simulink model "AutopilotLinear"  (R2021a)
settings: Solver=VariableStepAuto  StartTime=0.0  StopTime=2500  RelTol=1e-3
values from neighbouring files (symbols this model uses):
  A_final = [A1_long,zeros(5);zeros(5),A1_latr]    [runMeFirst.m]
  B_final = [B1_long,zeros(5,2);zeros(5,2),B1_latr]    [runMeFirst.m]
  C_final = [C1_long,zeros(5);zeros(5),C1_latr]    [runMeFirst.m]
  D_final = zeros(10,4)    [runMeFirst.m]
  Initial_h = 1000    [runMeFirst.m]
  K_deltas = [K_deltas_long,zeros(2);zeros(2),K_deltas_latr]    [runMeFirst.m]
  K_eps = [K_eps_long,zeros(2,2);zeros(2,2),K_eps_latr]    [runMeFirst.m]
  K_lqr = [K_lqr_long,zeros(2,5);zeros(2,5),K_lqr_latr]    [runMeFirst.m]
  Second_h = 2000    [runMeFirst.m]
  Start_time = 500    [runMeFirst.m]
  Start_turn = 1500    [runMeFirst.m]
  Step_timeh = 1000    [runMeFirst.m]
  T_a = 0.0495    [Auto_latr2.mat]
  T_e = 0.1    [Auto_long2.mat]
  T_p = 3.5    [Auto_long2.mat]
  T_r = 0.0495    [Auto_latr2.mat]
  Ue = 67    [runMeFirst.m]
undefined symbols (not defined in the file or in its folder): Des_rate, Des_roll
libraries: aerolibconvert2 x5, simulink x2
settings Model: Creator=panch  LastModifiedBy=panch

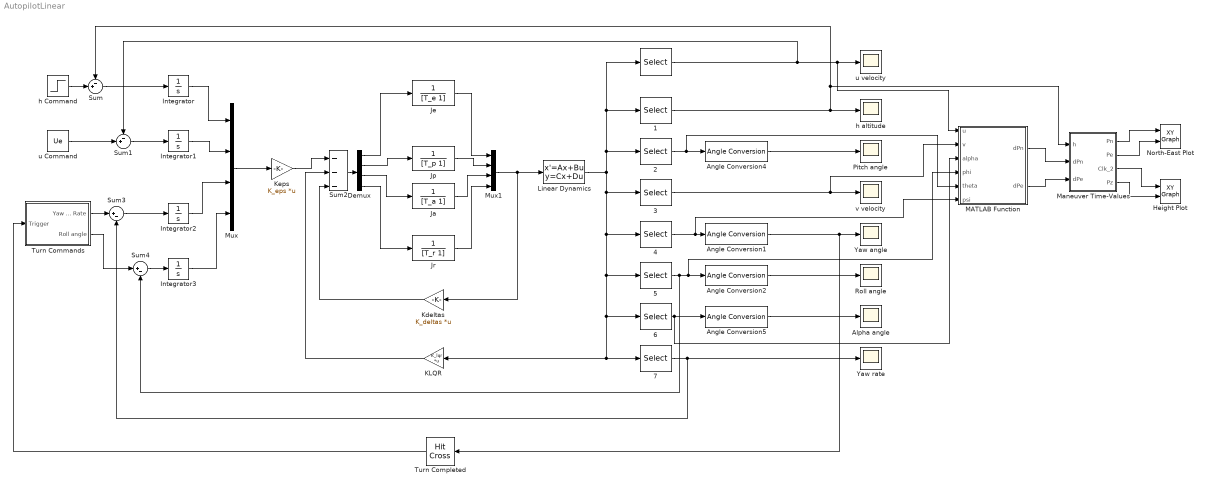
== system AutopilotLinear ==
  " " : Selector  InputPortWidth=10  IndexOptions=Index vector (dialog)  Indices=1  OutputSizes=1
  " 1" : Selector  InputPortWidth=10  IndexOptions=Index vector (dialog)  Indices=5  OutputSizes=1
  " 2" : Selector  InputPortWidth=10  IndexOptions=Index vector (dialog)  Indices=4  OutputSizes=1
  " 3" : Selector  InputPortWidth=10  IndexOptions=Index vector (dialog)  Indices=6  OutputSizes=1
  " 4" : Selector  InputPortWidth=10  IndexOptions=Index vector (dialog)  Indices=10  OutputSizes=1
  " 5" : Selector  InputPortWidth=10  IndexOptions=Index vector (dialog)  Indices=9  OutputSizes=1
  " 6" : Selector  InputPortWidth=10  IndexOptions=Index vector (dialog)  Indices=2  OutputSizes=1
  " 7" : Selector  InputPortWidth=10  IndexOptions=Index vector (dialog)  Indices=8  OutputSizes=1
  Alpha angle : Scope
  Angle Conversion{1..2,4..5} (4 alike) : aerolibconvert2/Angle Conversion  IU=rad  OU=deg
  Demux : Demux
  Height Plot : simulink/Sinks/XY Graph  xmin=0  xmax=2000  ymin=0  ymax=2500  st=-1
  Integrator{,1..3} (4 alike) : Integrator
  Ja : TransferFcn  Denominator=[T_a 1]
  Je : TransferFcn  Denominator=[T_e 1]
  Jp : TransferFcn  Denominator=[T_p 1]
  Jr : TransferFcn  Denominator=[T_r 1]
  KLQR : Gain  Gain=K_lqr  Multiplication=Matrix(K*u)
  Kdeltas : Gain  Gain=K_deltas  Multiplication=Matrix(K*u)
  Keps : Gain  Gain=K_eps  Multiplication=Matrix(K*u)
  Linear Dynamics : StateSpace  A=A_final  B=B_final  C=C_final  D=D_final  InitialCondition=0
  MATLAB Function : MATLAB Function  TreatAsAtomicUnit=on
  Maneuver Time-Values : Subsystem
  Mux : Mux
  Mux1 : Mux
  North-East Plot : simulink/Sinks/XY Graph  xmin=0  xmax=0.7e5  ymin=-100  ymax=4500  st=-1
  Pitch angle : Scope
  Roll angle : Scope
  Sum : Sum  Inputs=-+|
  Sum1 : Sum  Inputs=-+|
  Sum2 : Sum  Inputs=|---
  Sum3 : Sum  Inputs=|+-
  Sum4 : Sum  Inputs=|+-
  Turn Commands : Subsystem
  Turn Completed : HitCross  HitCrossingOffset=Yaw_des
  Yaw angle : Scope
  Yaw rate : Scope
  h Command : Step  Time=Step_timeh  Before=Initial_h  After=Second_h  SampleTime=0
  h altitude : Scope
  u Command : Constant  Value=Ue
  u velocity : Scope
  v velocity : Scope
  wires:
  Sum1/1 -> Integrator1/1
  Demux/2 -> Jp/1
  Mux/1 -> Keps/1
  Integrator/1 -> Mux/1
  h Command/1 -> Sum/2
  Jp/1 -> Mux1/2
  Sum2/1 -> Demux/1
  Demux/1 -> Je/1
  Keps/1 -> Sum2/1
  Integrator1/1 -> Mux/2
  Je/1 -> Mux1/1
  Sum/1 -> Integrator/1
  u Command/1 -> Sum1/2
  Demux/3 -> Ja/1
  Demux/4 -> Jr/1
  Ja/1 -> Mux1/3
  Jr/1 -> Mux1/4
  Mux1/1 -> Kdeltas/1, Linear Dynamics/1
  Kdeltas/1 -> Sum2/3
  KLQR/1 -> Sum2/2
  Linear Dynamics/1 -> " 2"/1, " 1"/1, " "/1, " 3"/1, " 4"/1, " 7"/1, KLQR/1, " 6"/1, " 5"/1
  " 3"/1 -> MATLAB Function/2(v), v velocity/1
  Angle Conversion4/1 -> Pitch angle/1
  " "/1 -> MATLAB Function/1(u), u velocity/1, Sum1/1
  " 1"/1 -> Maneuver Time-Values/1(h), Sum/1, h altitude/1
  Angle Conversion2/1 -> Roll angle/1
  " 5"/1 -> MATLAB Function/4(phi), Angle Conversion2/1, Sum4/2
  Angle Conversion1/1 -> Yaw angle/1, Turn Completed/1
  " 2"/1 -> MATLAB Function/5(theta), Angle Conversion4/1
  " 4"/1 -> MATLAB Function/6(psi), Angle Conversion1/1
  " 6"/1 -> Angle Conversion5/1, MATLAB Function/3(alpha)
  Sum4/1 -> Integrator3/1
  Sum3/1 -> Integrator2/1
  Integrator2/1 -> Mux/3
  Integrator3/1 -> Mux/4
  " 7"/1 -> Sum3/2, Yaw rate/1
  Angle Conversion5/1 -> Alpha angle/1
  MATLAB Function/1(dPn) -> Maneuver Time-Values/2(dPn)
  MATLAB Function/2(dPe) -> Maneuver Time-Values/3(dPe)
  Maneuver Time-Values/1(Pn) -> North-East Plot/1
  Maneuver Time-Values/2(Pe) -> North-East Plot/2
  Maneuver Time-Values/3(Clk_2) -> Height Plot/1
  Maneuver Time-Values/4(Pz) -> Height Plot/2
  Turn Completed/1 -> Turn Commands/1(Trigger)
  Turn Commands/1(Yaw Turn Rate) -> Sum3/1
  Turn Commands/2(Roll angle) -> Sum4/1

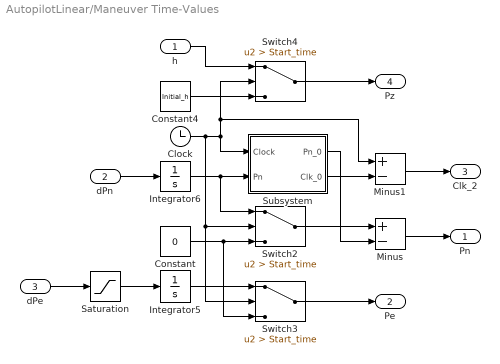
== system AutopilotLinear/Maneuver Time-Values ==
  h : Inport
  dPn : Inport  Port=2
  dPe : Inport  Port=3
  Clock : Clock
  Constant : Constant  Value=0
  Constant4 : Constant  Value=Initial_h
  Integrator5 : Integrator  ZeroCross=off
  Integrator6 : Integrator
  Minus : Sum  Inputs=+-
  Minus1 : Sum  Inputs=+-
  Saturation : Saturate  UpperLimit=inf  LowerLimit=0
  Subsystem : Subsystem
  Switch2 : Switch  Criteria=u2 > Threshold  Threshold=Start_time
  Switch3 : Switch  Criteria=u2 > Threshold  Threshold=Start_time
  Switch4 : Switch  Criteria=u2 > Threshold  Threshold=Start_time
  Pn : Outport
  Pe : Outport  Port=2
  Clk_2 : Outport  Port=3
  Pz : Outport  Port=4
  wires:
  Constant4/1 -> Switch4/3
  Switch2/1 -> Minus/1
  Switch4/1 -> Pz/1
  h/1 -> Switch4/1
  Switch3/1 -> Pe/1
  Constant/1 -> Switch2/3, Switch3/3
  Minus1/1 -> Clk_2/1
  dPe/1 -> Saturation/1
  Subsystem/2(Clk_0) -> Minus1/2
  Subsystem/1(Pn_0) -> Minus/2
  Integrator5/1 -> Switch3/1
  Saturation/1 -> Integrator5/1
  Minus/1 -> Pn/1
  dPn/1 -> Integrator6/1
  Clock/1 -> Switch3/2, Switch2/2, Minus1/1, Switch4/2, Subsystem/1(Clock)
  Integrator6/1 -> Switch2/1, Subsystem/2(Pn)

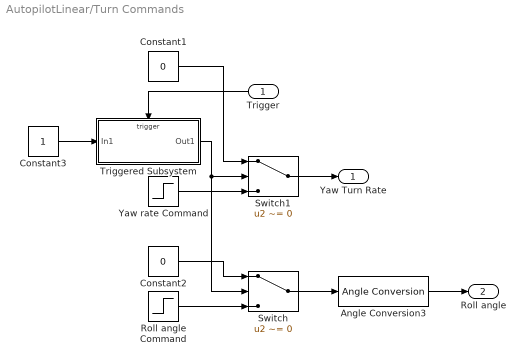
== system AutopilotLinear/Turn Commands ==
  Trigger : Inport
  Angle Conversion3 : aerolibconvert2/Angle Conversion  IU=deg  OU=rad
  Constant1 : Constant  Value=0
  Constant2 : Constant  Value=0
  Constant3 : Constant
  Roll angle Command : Step  Time=Start_turn  After=Des_roll  SampleTime=0
  Switch : Switch  Criteria=u2 ~= 0  Threshold=180  SaturateOnIntegerOverflow=on
  Switch1 : Switch  Criteria=u2 ~= 0  Threshold=180  SaturateOnIntegerOverflow=on
  Triggered Subsystem : Subsystem  TreatAsAtomicUnit=on
  Yaw rate Command : Step  Time=Start_turn  After=Des_rate  SampleTime=0
  Yaw Turn Rate : Outport
  Roll angle : Outport  Port=2
  wires:
  Angle Conversion3/1 -> Roll angle/1
  Switch/1 -> Angle Conversion3/1
  Switch1/1 -> Yaw Turn Rate/1
  Yaw rate Command/1 -> Switch1/3
  Constant1/1 -> Switch1/1
  Constant3/1 -> Triggered Subsystem/1(In1)
  Roll angle Command/1 -> Switch/3
  Trigger/1 -> Triggered Subsystem/Trigger
  Constant2/1 -> Switch/1
  Triggered Subsystem/1(Out1) -> Switch/2, Switch1/2

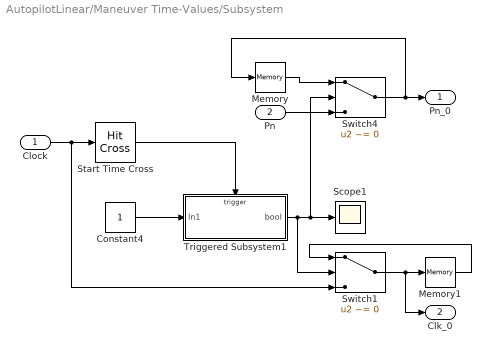
== system AutopilotLinear/Maneuver Time-Values/Subsystem ==
  Clock : Inport
  Pn : Inport  Port=2
  Constant4 : Constant
  Memory : Memory  InheritSampleTime=on
  Memory1 : Memory  InheritSampleTime=on
  Scope1 : Scope
  Start Time Cross : HitCross  HitCrossingOffset=Start_time
  Switch1 : Switch  Criteria=u2 ~= 0
  Switch4 : Switch  Criteria=u2 ~= 0
  Triggered Subsystem1 : Subsystem  TreatAsAtomicUnit=on
  Pn_0 : Outport
  Clk_0 : Outport  Port=2
  wires:
  Switch1/1 -> Memory1/1, Clk_0/1
  Constant4/1 -> Triggered Subsystem1/1(In1)
  Memory1/1 -> Switch1/1
  Memory/1 -> Switch4/1
  Triggered Subsystem1/1(bool) -> Switch4/2, Scope1/1, Switch1/2
  Start Time Cross/1 -> Triggered Subsystem1/Trigger
  Pn/1 -> Switch4/3
  Clock/1 -> Start Time Cross/1, Switch1/3
  Switch4/1 -> Memory/1, Pn_0/1

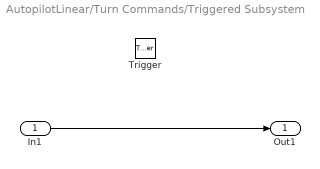
== system AutopilotLinear/Turn Commands/Triggered Subsystem ==
  In1 : Inport
  Trigger : TriggerPort  VariantControl=(inherit)
  Out1 : Outport
  wires:
  In1/1 -> Out1/1

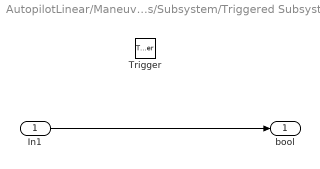
== system AutopilotLinear/Maneuver Time-Values/Subsystem/Triggered Subsystem1 ==
  In1 : Inport
  Trigger : TriggerPort  VariantControl=(inherit)
  bool : Outport
  wires:
  In1/1 -> bool/1

== matlab function AutopilotLinear/MATLAB Function ==
  data: u input; dPn output; v input; alpha input; phi input; theta input; psi input; dPe output
function [dPn,dPe] = inertia(u,v,alpha,phi,theta,psi)
% Funtion to compute North (x) and east (y) position.
w = alpha*u;
matrix = [cos(theta)*cos(psi),sin(phi)*sin(theta)*cos(psi)-cos(phi)*sin(psi),cos(phi)*sin(theta)*cos(psi)+sin(phi)*sin(psi);...
    cos(theta)*sin(psi), sin(phi)*sin(theta)*sin(psi)+cos(phi)*cos(psi),cos(phi)*sin(theta)*sin(psi)-sin(phi)*cos(psi)];
states = matrix*[u;v;w];
dPn = states(1);
dPe = states(2);
